simulink model "ExperimentalPowertrain"  (R2019b)
settings: Solver=ode1  StartTime=0.0  StopTime=inf  FixedStep=0.0002  RelTol=1e-3
PreLoadFcn:
  | vehicle = 'Car'; if ~length(which('cmself')), cmenv; end
  | ExperimentalPowertrain_bus
InitFcn:
  | vehicle = 'Car'; if ~length(which('cmself')), cmenv; end
  | ExperimentalPowertrain_bus
libraries: CarMaker4SL x8
(part 2 of 2)

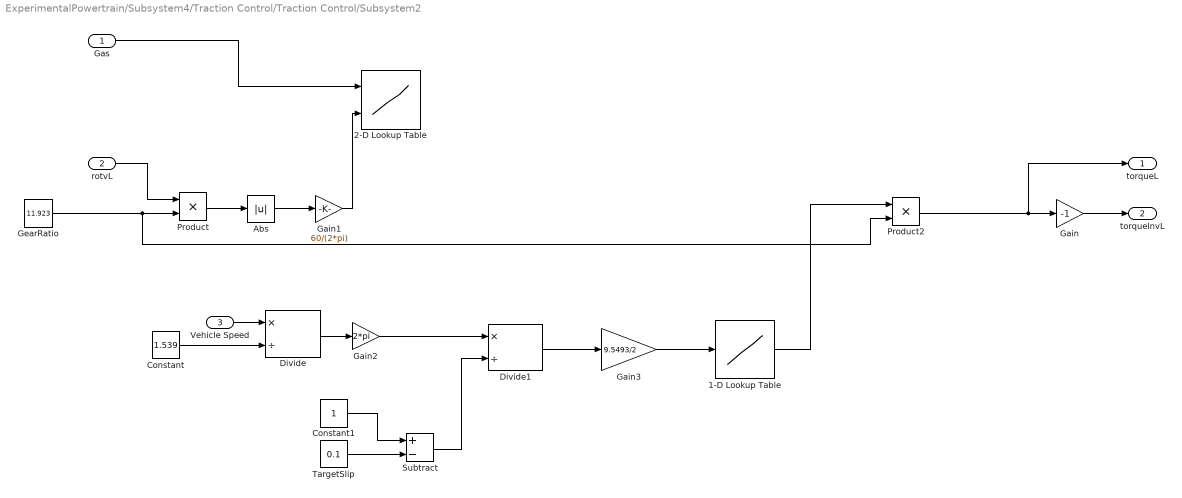
== system ExperimentalPowertrain/Subsystem4/Traction Control/Traction Control/Subsystem2 ==
  Gas : Inport
  rotvL : Inport  Port=2
  Vehicle Speed : Inport  Port=3
  1-D Lookup Table : Lookup_n-D  NumberOfTableDimensions=1  BreakpointsForDimension1=[0 2000 4000 6000 8000 10000 12000 14000 15000 16000 17000 18000 20000 22000]  Table=[21 21 21 21 21 21 21 21 21 20 20 19 15 0]  InternalRulePriority=Speed  RndMeth=Simplest  InputSameDT=on
  2-D Lookup Table : Lookup_n-D  BreakpointsForDimension1=[0 0.2 0.4 0.6 0.8 1]  BreakpointsForDimension2=[0 2000 4000 6000 8000 10000 12000 14000 15000 16000 17000 18000 20000 22000]  Table=[0 0 0 0 0 0 0 0 0 0 0 0 0 0;4 4 4 4 4 4 4 4 4 4 4 4 3 0;8 8 8 8 8 8 8 8 8 8 8 8 6 0;13 13 13 13 13 13 13 13 13 12 12 11 9 0;17 17 17 17 17 17 17 17 17 16 16 15 12 0;21 21 21 21 21 21 21 21 21 20 20 19 15 0]  InternalRulePriority=Speed  RndMeth=Simplest  InputSameDT=on
  Abs : Abs
  Constant : Constant  Value=1.539
  Constant1 : Constant
  Divide : Product  Inputs=*/
  Divide1 : Product  Inputs=*/
  Gain : Gain  Gain=-1
  Gain1 : Gain  Gain=60/(2*pi)
  Gain2 : Gain  Gain=2*pi
  Gain3 : Gain  Gain=9.5493/2
  GearRatio : Constant  Value=11.923
  Product : Product
  Product2 : Product
  Subtract : Sum  Inputs=+-
  TargetSlip : Constant  Value=0.1
  torqueL : Outport
  torqueInvL : Outport  Port=2
  wires:
  Gain/1 -> torqueInvL/1
  Product/1 -> Abs/1
  Gas/1 -> 2-D Lookup Table/1
  GearRatio/1 -> Product2/2, Product/2
  rotvL/1 -> Product/1
  Product2/1 -> Gain/1, torqueL/1
  Abs/1 -> Gain1/1
  Gain1/1 -> 2-D Lookup Table/2
  TargetSlip/1 -> Subtract/2
  Vehicle Speed/1 -> Divide/1
  Constant/1 -> Divide/2
  Divide/1 -> Gain2/1
  Gain2/1 -> Divide1/1
  Constant1/1 -> Subtract/1
  Subtract/1 -> Divide1/2
  Divide1/1 -> Gain3/1
  Gain3/1 -> 1-D Lookup Table/1
  1-D Lookup Table/1 -> Product2/1

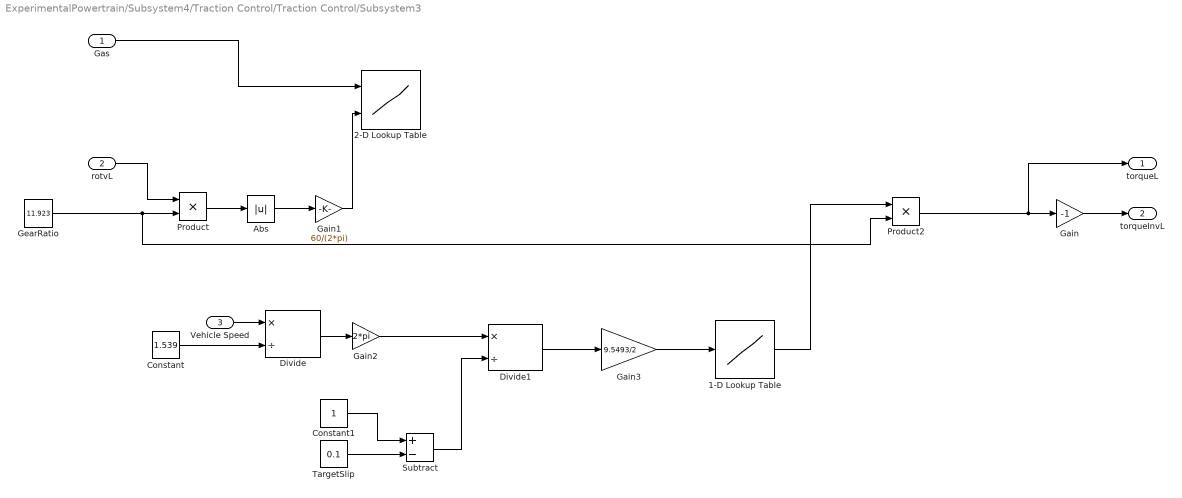
== system ExperimentalPowertrain/Subsystem4/Traction Control/Traction Control/Subsystem3 ==
  Gas : Inport
  rotvL : Inport  Port=2
  Vehicle Speed : Inport  Port=3
  1-D Lookup Table : Lookup_n-D  NumberOfTableDimensions=1  BreakpointsForDimension1=[0 2000 4000 6000 8000 10000 12000 14000 15000 16000 17000 18000 20000 22000]  Table=[21 21 21 21 21 21 21 21 21 20 20 19 15 0]  InternalRulePriority=Speed  RndMeth=Simplest  InputSameDT=on
  2-D Lookup Table : Lookup_n-D  BreakpointsForDimension1=[0 0.2 0.4 0.6 0.8 1]  BreakpointsForDimension2=[0 2000 4000 6000 8000 10000 12000 14000 15000 16000 17000 18000 20000 22000]  Table=[0 0 0 0 0 0 0 0 0 0 0 0 0 0;4 4 4 4 4 4 4 4 4 4 4 4 3 0;8 8 8 8 8 8 8 8 8 8 8 8 6 0;13 13 13 13 13 13 13 13 13 12 12 11 9 0;17 17 17 17 17 17 17 17 17 16 16 15 12 0;21 21 21 21 21 21 21 21 21 20 20 19 15 0]  InternalRulePriority=Speed  RndMeth=Simplest  InputSameDT=on
  Abs : Abs
  Constant : Constant  Value=1.539
  Constant1 : Constant
  Divide : Product  Inputs=*/
  Divide1 : Product  Inputs=*/
  Gain : Gain  Gain=-1
  Gain1 : Gain  Gain=60/(2*pi)
  Gain2 : Gain  Gain=2*pi
  Gain3 : Gain  Gain=9.5493/2
  GearRatio : Constant  Value=11.923
  Product : Product
  Product2 : Product
  Subtract : Sum  Inputs=+-
  TargetSlip : Constant  Value=0.1
  torqueL : Outport
  torqueInvL : Outport  Port=2
  wires:
  Gain/1 -> torqueInvL/1
  Product/1 -> Abs/1
  Gas/1 -> 2-D Lookup Table/1
  GearRatio/1 -> Product2/2, Product/2
  rotvL/1 -> Product/1
  Product2/1 -> Gain/1, torqueL/1
  Abs/1 -> Gain1/1
  Gain1/1 -> 2-D Lookup Table/2
  TargetSlip/1 -> Subtract/2
  Vehicle Speed/1 -> Divide/1
  Constant/1 -> Divide/2
  Divide/1 -> Gain2/1
  Gain2/1 -> Divide1/1
  Constant1/1 -> Subtract/1
  Subtract/1 -> Divide1/2
  Divide1/1 -> Gain3/1
  Gain3/1 -> 1-D Lookup Table/1
  1-D Lookup Table/1 -> Product2/1

== system ExperimentalPowertrain/Subsystem4/Launch Control/LaunchControl/Subsystem/If Action Subsystem ==
  In1 : Inport
  Action Port : ActionPort  ActionPortLabel=if(u2< u1)
  Out1 : Outport
  wires:
  In1/1 -> Out1/1

== system ExperimentalPowertrain/Subsystem4/Launch Control/LaunchControl/Subsystem/If Action Subsystem1 ==
  In1 : Inport
  Action Port : ActionPort  ActionPortLabel=else
  Out1 : Outport
  wires:
  In1/1 -> Out1/1

== system ExperimentalPowertrain/Subsystem4/Launch Control/LaunchControl/Subsystem1/If Action Subsystem ==
  In1 : Inport
  Action Port : ActionPort  ActionPortLabel=if(u2< u1)
  Out1 : Outport
  wires:
  In1/1 -> Out1/1

== system ExperimentalPowertrain/Subsystem4/Launch Control/LaunchControl/Subsystem1/If Action Subsystem1 ==
  In1 : Inport
  Action Port : ActionPort  ActionPortLabel=else
  Out1 : Outport
  wires:
  In1/1 -> Out1/1

== system ExperimentalPowertrain/Subsystem4/Launch Control/LaunchControl/Subsystem2/If Action Subsystem ==
  In1 : Inport
  Action Port : ActionPort  ActionPortLabel=if(u2< u1)
  Out1 : Outport
  wires:
  In1/1 -> Out1/1

== system ExperimentalPowertrain/Subsystem4/Launch Control/LaunchControl/Subsystem2/If Action Subsystem1 ==
  In1 : Inport
  Action Port : ActionPort  ActionPortLabel=else
  Out1 : Outport
  wires:
  In1/1 -> Out1/1

== system ExperimentalPowertrain/Subsystem4/Launch Control/LaunchControl/Subsystem3/If Action Subsystem ==
  In1 : Inport
  Action Port : ActionPort  ActionPortLabel=if(u2< u1)
  Out1 : Outport
  wires:
  In1/1 -> Out1/1

== system ExperimentalPowertrain/Subsystem4/Launch Control/LaunchControl/Subsystem3/If Action Subsystem1 ==
  In1 : Inport
  Action Port : ActionPort  ActionPortLabel=else
  Out1 : Outport
  wires:
  In1/1 -> Out1/1
